simulink model "myexp8"  (R2022a)
settings: Solver=VariableStepAuto  StartTime=0.0  StopTime=10  RelTol=1e-3
values from neighbouring files (symbols this model uses):
  k = k_list(i)    [exp8.m]
  M = M_list(i)    [exp8.m]
libraries: commdigbbndpm3 x3, commchan3 x2, commsink2 x2, commrandsrc3 x1, commfilt2 x1, dspstat3 x1, dspsigops x1
settings Model: Creator=惠普  LastModifiedBy=惠普

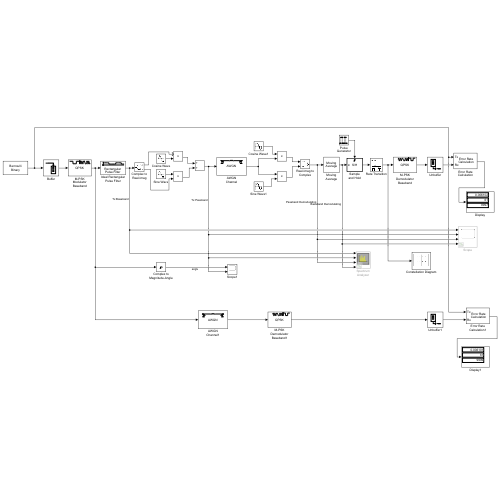
[thumbnail: Simulink's stored preview of the top-level diagram]
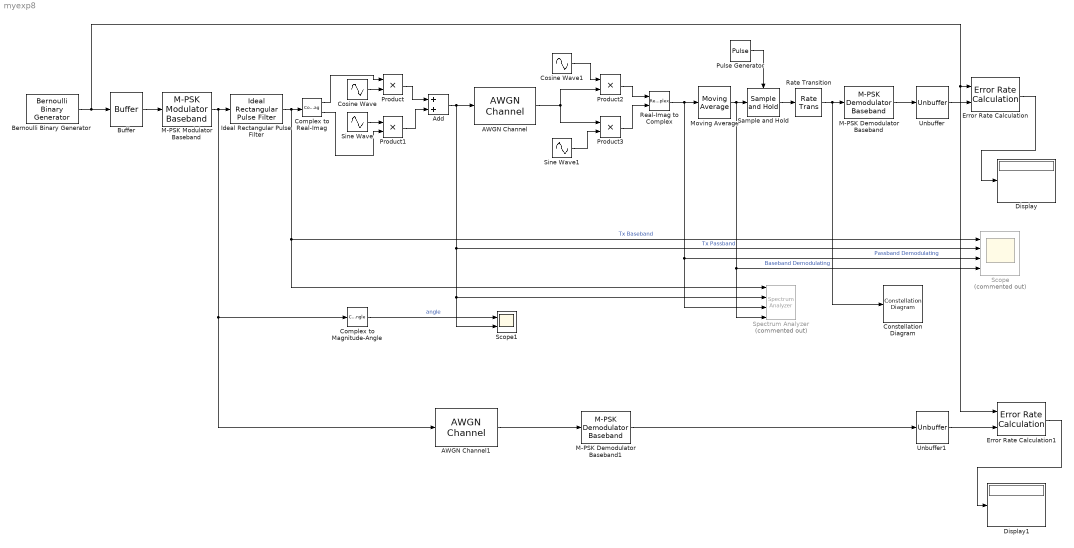
== system myexp8 ==
  AWGN Channel : commchan3/AWGN Channel  InputProcessing=Columns as channels (frame based)  seed=137  noiseMode="Signal to noise ratio  (Eb/No)"  EbNodB=5  EsNodB=10  SNRdB=10  bitsPerSym=k  Ps=1  Tsym=k*1e-3  variance=1
  AWGN Channel1 : commchan3/AWGN Channel  InputProcessing=Columns as channels (frame based)  seed=137  noiseMode="Signal to noise ratio  (Eb/No)"  EbNodB=5  EsNodB=10  SNRdB=10  bitsPerSym=k  Ps=1  Tsym=k*1e-3  variance=1
  Add : Sum
  Bernoulli Binary Generator : commrandsrc3/Bernoulli Binary Generator  ProbabilityOfZero=0.5  SeedSource=Auto  Seed=0  SampleTime=1e-3  SamplesPerFrame=1  OutputDataType=double  SimulateUsing=Interpreted execution
  Buffer : Buffer  N=k  OutputFrames=off
  Complex to Magnitude-Angle : ComplexToMagnitudeAngle  Output=Angle
  Complex to Real-Imag : ComplexToRealImag
  Constellation Diagram : ConstellationDiagram  WindowPosition=[128.000000,126.000000,600.000000,586.000000,]  ScopeFrameLocation=window  SymbolsToDisplaySource=Property  SymbolsToDisplay=100  XLimits=[-1.49,1.49]  YLimits=[-1.38,1.38]
  Cosine Wave : Sin  Amplitude=sqrt(2)  Frequency=2*pi*(10e3)  Phase=pi/2  SampleTime=1e-6
  Cosine Wave1 : Sin  Amplitude=sqrt(2)  Frequency=2*pi*(10e3)  Phase=pi/2  SampleTime=1e-6
  Display : Display
  Display1 : Display
  Error Rate Calculation : commsink2/Error Rate Calculation  N=2*k  st_delay=0  cp_mode=Entire frame  subframe=[]  PMode=Port  WsName=ErrorVec  RsMode2=off  stop=off  numErr=100  maxBits=1e6
  Error Rate Calculation1 : commsink2/Error Rate Calculation  N=k  st_delay=0  cp_mode=Entire frame  subframe=[]  PMode=Port  WsName=ErrorVec  RsMode2=off  stop=off  numErr=100  maxBits=1e6
  Ideal Rectangular Pulse Filter : commfilt2/Ideal Rectangular Pulse Filter  pulseLen=k*1000  pulseDelay=0  InputProcessing=Columns as channels (frame based)  RateOptions=Allow multirate processing  sampMode=Mute  normCheck=off  normMode=Sum of samples  filterGain=1  saveAsFlag=0  roundingMode=Floor  overflowMode=off  firstCoeffDataTypeStr=Inherit: Same word length as input  firstCoeffMin=[]  firstCoeffMax=[]  firstCoeffLastDataTypeStr=Inherit: Same word length as input  outputDataTypeStr=Inherit: Same as accumulator  outputMin=[]  outputMax=[]  outputLastDataTypeStr=Inherit: Same as accumulator
      settings: SourceProductBaseCode=CM
  M-PSK Demodulator Baseband : commdigbbndpm3/M-PSK Demodulator Baseband  M=M  OutType=Bit  DecType=Hard decision  VarSource=Dialog  Variance=1  Dec=Gray  Mapping=[0:7]  Ph=pi/M  outDtype1=Inherit via internal rule  outDtype2=Inherit via internal rule  derotateFactorWordLen=16  derotateFactorDataTypeStr=Inherit: Same word length as input  derotateFactorLastDataTypeStr=Inherit: Same word length as input
  M-PSK Demodulator Baseband1 : commdigbbndpm3/M-PSK Demodulator Baseband  M=M  OutType=Bit  DecType=Hard decision  VarSource=Dialog  Variance=1  Dec=Gray  Mapping=[0:7]  Ph=pi/M  outDtype1=Inherit via internal rule  outDtype2=Inherit via internal rule  derotateFactorWordLen=16  derotateFactorDataTypeStr=Inherit: Same word length as input  derotateFactorLastDataTypeStr=Inherit: Same word length as input
  M-PSK Modulator Baseband : commdigbbndpm3/M-PSK Modulator Baseband  M=M  InType=Bit  Enc=Gray  Mapping=[0:7]  Ph=pi/M  outDtype=double  outWordLen=16  outUDDataType=sfix(16)  outFracLenMode=Best precision  outFracLen=15  outDataTypeStr=double  outLastDataTypeStr=double
  Moving Average : dspstat3/Moving Average  Method=Sliding window  ForgettingFactorPort=off  SpecifyWindowLength=on  WindowLength=k*1e3  ForgettingFactor=0.9  SimulateUsing=Code generation
  Product{,1..3} (4 alike) : Product
  Pulse Generator : DiscretePulseGenerator  Period=k*1e3  SampleTime=1e-6
  Rate Transition : RateTransition  OutPortSampleTime=k*1e-3
  Real-Imag to Complex : RealImagToComplex
  Sample and Hold : dspsigops/Sample and Hold  trig=Rising edge  initCond=0  latchinput=off
  Scope : Scope  Commented=on  NumInputPorts=4
  Scope1 : Scope  NumInputPorts=2
  Sine Wave : Sin  Amplitude=sqrt(2)  Frequency=2*pi*(10e3)  Phase=pi  SampleTime=1e-6
  Sine Wave1 : Sin  Amplitude=sqrt(2)  Frequency=2*pi*(10e3)  Phase=pi  SampleTime=1e-6
  Spectrum Analyzer : SpectrumAnalyzer  Commented=on  NumInputPorts=4
  Unbuffer : Unbuffer
  Unbuffer1 : Unbuffer
  wires:
  Bernoulli Binary Generator/1 -> Error Rate Calculation1/1, Error Rate Calculation/1, Buffer/1
  Buffer/1 -> M-PSK Modulator Baseband/1
  M-PSK Modulator Baseband/1 -> AWGN Channel1/1, Complex to Magnitude-Angle/1, Ideal Rectangular Pulse Filter/1
  Ideal Rectangular Pulse Filter/1 -> Spectrum Analyzer/1, Scope/1, Complex to Real-Imag/1  "Tx Baseband"
  Sine Wave/1 -> Product1/1
  Complex to Real-Imag/2 -> Product1/2
  Cosine Wave/1 -> Product/2
  Complex to Real-Imag/1 -> Product/1
  Product/1 -> Add/1
  Product1/1 -> Add/2
  Add/1 -> Scope1/2, Spectrum Analyzer/2, Scope/2, AWGN Channel/1  "Tx Passband"
  Product2/1 -> Real-Imag to Complex/1
  Product3/1 -> Real-Imag to Complex/2
  AWGN Channel/1 -> Product3/1, Product2/2
  Cosine Wave1/1 -> Product2/1
  Sine Wave1/1 -> Product3/2
  Real-Imag to Complex/1 -> Moving Average/1, Spectrum Analyzer/3, Scope/3  "Passband Demodulating"
  Moving Average/1 -> Spectrum Analyzer/4, Scope/4, Sample and Hold/1  "Baseband Demodulating"
  Pulse Generator/1 -> Sample and Hold/Trigger
  Sample and Hold/1 -> Rate Transition/1
  Rate Transition/1 -> Constellation Diagram/1, M-PSK Demodulator Baseband/1
  M-PSK Demodulator Baseband/1 -> Unbuffer/1
  Unbuffer/1 -> Error Rate Calculation/2
  Error Rate Calculation/1 -> Display/1
  Complex to Magnitude-Angle/1 -> Scope1/1  "angle"
  AWGN Channel1/1 -> M-PSK Demodulator Baseband1/1
  Error Rate Calculation1/1 -> Display1/1
  M-PSK Demodulator Baseband1/1 -> Unbuffer1/1
  Unbuffer1/1 -> Error Rate Calculation1/2
